simulink model "RobustLateralLPV"  (R2020b)
settings: Solver=VariableStepAuto  StartTime=0.0  StopTime=64  RelTol=1e-3
values from neighbouring files (symbols this model uses):
  A11 = [-(Cf + Cr)/(m*vxmax)        -vxmin + (Cr*Lr - Cf*Lf)/(m*vxmax) ... (first row only)    [Lab_Lateral.m]
  A12 = [-(Cf + Cr)/(m*vxmin)        -vxmin + (Cr*Lr - Cf*Lf)/(m*vxmin) ... (first row only)    [Lab_Lateral.m]
  A21 = [-(Cf + Cr)/(m*vxmax)        -vxmax + (Cr*Lr - Cf*Lf)/(m*vxmax) ... (first row only)    [Lab_Lateral.m]
  A22 = [-(Cf + Cr)/(m*vxmin)        -vxmax + (Cr*Lr - Cf*Lf)/(m*vxmin) ... (first row only)    [Lab_Lateral.m]
  B = [Cf/m; Lf*Cf/Iz]    [Lab_Lateral.m]
  C = [0 1]    [Lab_Lateral.m]
  D = [0]    [Lab_Lateral.m]
  listG = {G1, G2, G3, G4}    [H_inf_control_designLPV.m]
  listK = {K1, K2, K3, K4}    [H_inf_control_designLPV.m]
  m = 1621    [Lab_Lateral.m]
  rho1Max = vxmax    (= 15)    [Lab_Lateral.m]
  rho1Min = vxmin    (= 5)    [Lab_Lateral.m]
  rho2Max = 1/vxmin    (= 0.2)    [Lab_Lateral.m]
  rho2Min = 1/vxmax    (= 0.0666666666667)    [Lab_Lateral.m]
libraries: simulink x4, cstblocks x1
settings Model: Creator=DELL  LastModifiedBy=DELL

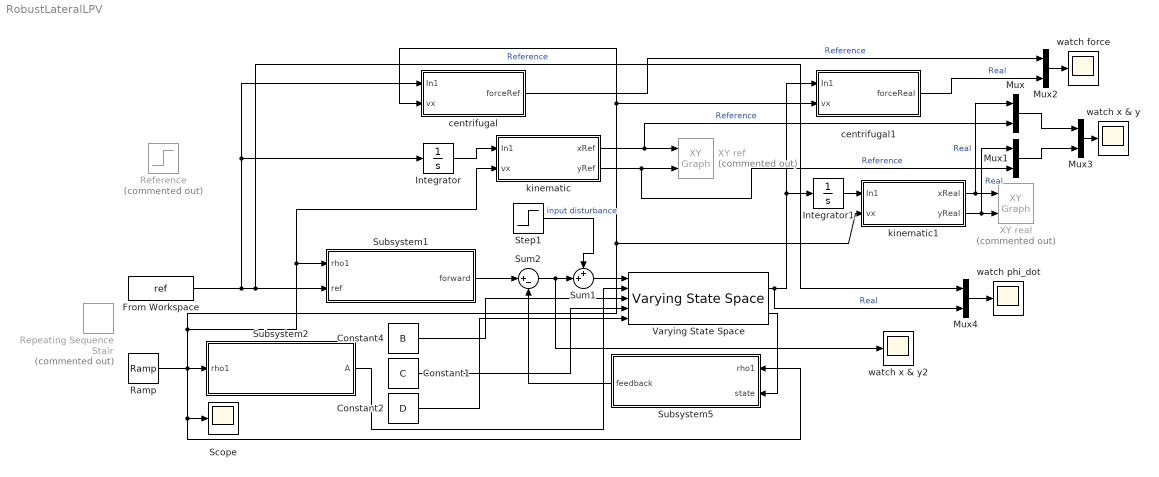
== system RobustLateralLPV ==
  Constant1 : Constant  Value=C  VectorParams1D=off
  Constant2 : Constant  Value=D
  Constant4 : Constant  Value=B
  From Workspace : FromWorkspace  VariableName=ref
  Integrator : Integrator
  Integrator1 : Integrator
  Mux{,1..4} (5 alike) : Mux  Inputs=2
  Ramp : simulink/Sources/Ramp  slope=0.2  start=20  InitialOutput=5
  Reference : Step  Commented=on  SampleTime=0
  Repeating Sequence Stair : simulink/Sources/Repeating Sequence Stair  Commented=on  OutValues=[5 11 15 9 7 5].'  tsamp=10  OutMin=[]  OutMax=[]  OutDataTypeStr=double  OutputDataTypeScalingMode=double  OutDataType=fixdt(0,8)  ConRadixGroup=Best Precision: Vector-wise  OutScaling=2^-12
  Scope : Scope
  Step1 : Step  Time=2  After=0.02*0  SampleTime=0
  Subsystem1 : Subsystem
  Subsystem2 : Subsystem
  Subsystem5 : Subsystem
  Sum1 : Sum  Inputs=++|
  Sum2 : Sum  Inputs=|+-
  Varying State Space : cstblocks/Linear Parameter Varying/Varying State Space  x0=0  xNames=''  OutputX=on  OutputDX=off
  XY real : simulink/Sinks/XY Graph  Commented=on  xmin=0  xmax=400  ymin=0  ymax=350  st=ts
  XY ref : simulink/Sinks/XY Graph  Commented=on  xmin=0  xmax=400  ymin=0  ymax=350  st=ts
  centrifugal : Subsystem
  centrifugal1 : Subsystem
  kinematic : Subsystem
  kinematic1 : Subsystem
  watch force : Scope
  watch phi_dot : Scope
  watch x & y : Scope
  watch x & y2 : Scope
  wires:
  Sum1/1 -> Varying State Space/1
  Mux/1 -> Mux3/1
  kinematic/1(xRef) -> Mux/2, XY ref/1  "Reference"
  Integrator/1 -> kinematic/1(In1)
  Integrator1/1 -> kinematic1/1(In1)
  Varying State Space/1 -> Mux4/2, centrifugal1/1(In1), Integrator1/1  "Real"
  centrifugal1/1(forceReal) -> Mux2/2  "Real"
  Sum2/1 -> watch x & y2/1, Sum1/2
  kinematic/2(yRef) -> Mux1/2, XY ref/2  "Reference"
  Step1/1 -> Sum1/1  "input disturbance"
  kinematic1/2(yReal) -> Mux1/1, XY real/2  "Real"
  centrifugal/1(forceRef) -> Mux2/1  "Reference"
  kinematic1/1(xReal) -> Mux/1, XY real/1  "Real"
  Subsystem1/1(forward) -> Sum2/1
  Subsystem5/1(feedback) -> Sum2/2
  Mux1/1 -> Mux3/2
  From Workspace/1 -> centrifugal/1(In1), Integrator/1, Mux4/1, Subsystem1/2(ref)  "Reference"
  Varying State Space/2 -> Subsystem5/2(state)
  Constant4/1 -> Varying State Space/3
  Constant1/1 -> Varying State Space/4
  Constant2/1 -> Varying State Space/5
  Ramp/1 -> Subsystem2/1(rho1), kinematic/2(vx), Subsystem1/1(rho1), centrifugal/2(vx), centrifugal1/2(vx), kinematic1/2(vx), Subsystem5/1(rho1), Scope/1
  Subsystem2/1(A) -> Varying State Space/2
  Mux4/1 -> watch phi_dot/1
  Mux3/1 -> watch x & y/1
  Mux2/1 -> watch force/1

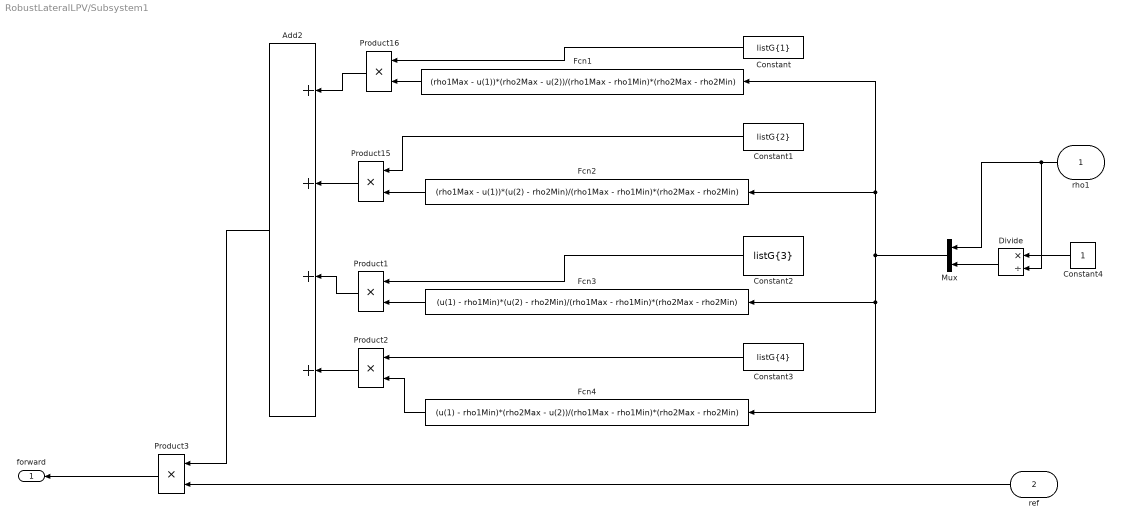
== system RobustLateralLPV/Subsystem1 ==
  rho1 : Inport
  ref : Inport  Port=2
  Add2 : Sum  Inputs=++++
  Constant : Constant  Value=listG{1}
  Constant1 : Constant  Value=listG{2}
  Constant2 : Constant  Value=listG{3}
  Constant3 : Constant  Value=listG{4}
  Constant4 : Constant
  Divide : Product  Inputs=*/
  Fcn1 : Fcn  Expr=(rho1Max - u(1))*(rho2Max - u(2))/(rho1Max - rho1Min)*(rho2Max - rho2Min)
  Fcn2 : Fcn  Expr=(rho1Max - u(1))*(u(2) - rho2Min)/(rho1Max - rho1Min)*(rho2Max - rho2Min)
  Fcn3 : Fcn  Expr=(u(1) - rho1Min)*(u(2) - rho2Min)/(rho1Max - rho1Min)*(rho2Max - rho2Min)
  Fcn4 : Fcn  Expr=(u(1) - rho1Min)*(rho2Max - u(2))/(rho1Max - rho1Min)*(rho2Max - rho2Min)
  Mux : Mux  Inputs=2
  Product{1..3,15..16} (5 alike) : Product  RndMeth=Zero
  forward : Outport  VectorParamsAs1DForOutWhenUnconnected=off
  wires:
  Fcn1/1 -> Product16/2
  Fcn2/1 -> Product15/2
  Product16/1 -> Add2/1
  Product15/1 -> Add2/2
  Constant1/1 -> Product15/1
  Constant/1 -> Product16/1
  rho1/1 -> Divide/2, Mux/1
  Mux/1 -> Fcn4/1, Fcn3/1, Fcn1/1, Fcn2/1
  Fcn3/1 -> Product1/2
  Constant2/1 -> Product1/1
  Product1/1 -> Add2/3
  Product2/1 -> Add2/4
  Fcn4/1 -> Product2/2
  Constant3/1 -> Product2/1
  Product3/1 -> forward/1
  Add2/1 -> Product3/1
  ref/1 -> Product3/2
  Divide/1 -> Mux/2
  Constant4/1 -> Divide/1

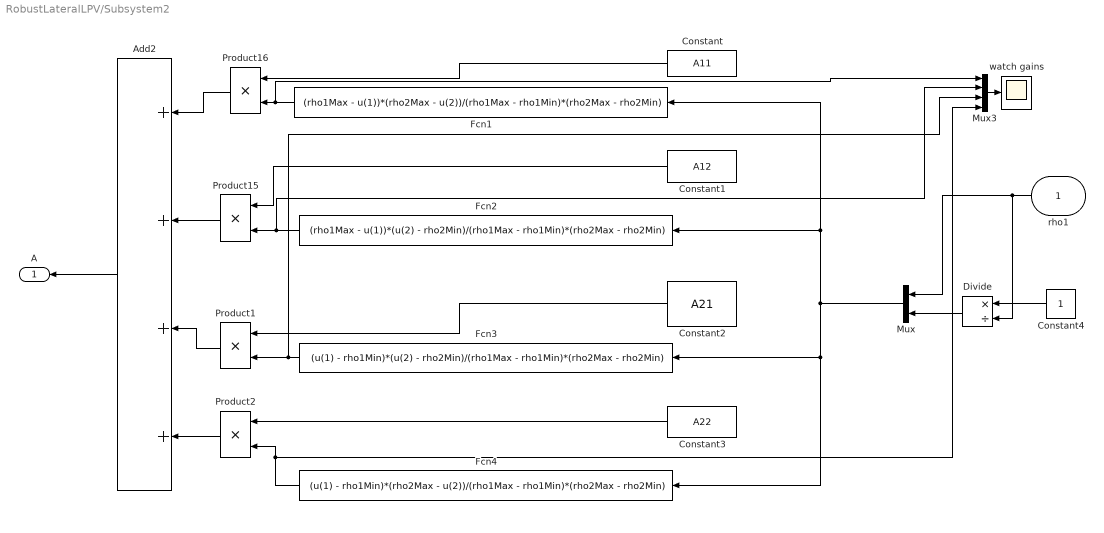
== system RobustLateralLPV/Subsystem2 ==
  rho1 : Inport
  Add2 : Sum  Inputs=++++
  Constant : Constant  Value=A11
  Constant1 : Constant  Value=A12
  Constant2 : Constant  Value=A21
  Constant3 : Constant  Value=A22
  Constant4 : Constant
  Divide : Product  Inputs=*/
  Fcn1 : Fcn  Expr=(rho1Max - u(1))*(rho2Max - u(2))/(rho1Max - rho1Min)*(rho2Max - rho2Min)
  Fcn2 : Fcn  Expr=(rho1Max - u(1))*(u(2) - rho2Min)/(rho1Max - rho1Min)*(rho2Max - rho2Min)
  Fcn3 : Fcn  Expr=(u(1) - rho1Min)*(u(2) - rho2Min)/(rho1Max - rho1Min)*(rho2Max - rho2Min)
  Fcn4 : Fcn  Expr=(u(1) - rho1Min)*(rho2Max - u(2))/(rho1Max - rho1Min)*(rho2Max - rho2Min)
  Mux : Mux  Inputs=2
  Mux3 : Mux
  Product{1..2,15..16} (4 alike) : Product  RndMeth=Zero
  watch gains : Scope
  A : Outport  VectorParamsAs1DForOutWhenUnconnected=off
  wires:
  Fcn1/1 -> Mux3/1, Product16/2
  Fcn2/1 -> Mux3/2, Product15/2
  Product15/1 -> Add2/2
  Constant1/1 -> Product15/1
  Constant/1 -> Product16/1
  rho1/1 -> Divide/2, Mux/1
  Mux/1 -> Fcn4/1, Fcn3/1, Fcn1/1, Fcn2/1
  Constant2/1 -> Product1/1
  Product1/1 -> Add2/3
  Product2/1 -> Add2/4
  Fcn4/1 -> Mux3/4, Product2/2
  Constant3/1 -> Product2/1
  Divide/1 -> Mux/2
  Constant4/1 -> Divide/1
  Add2/1 -> A/1
  Mux3/1 -> watch gains/1
  Fcn3/1 -> Product1/2, Mux3/3
  Product16/1 -> Add2/1

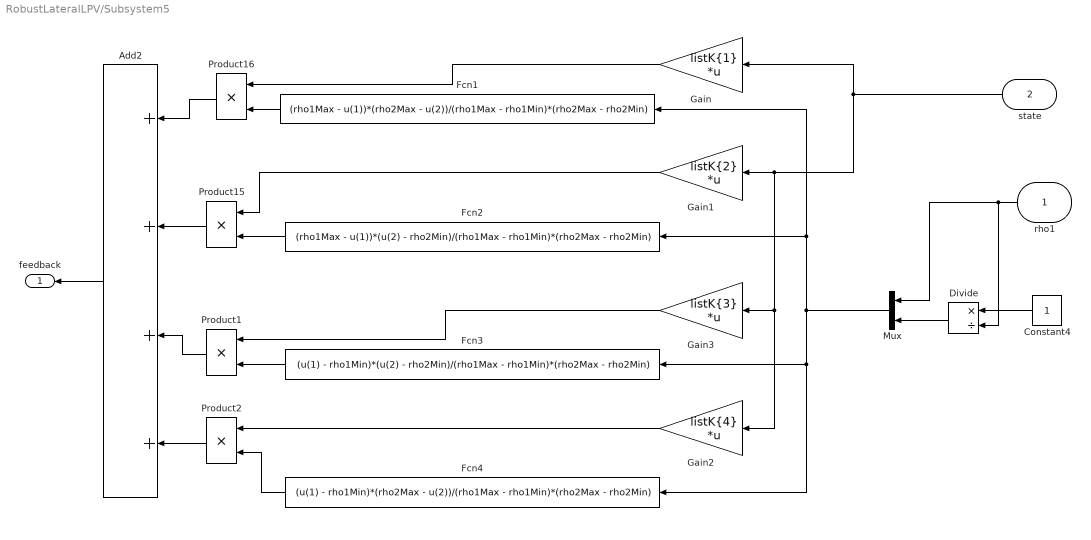
== system RobustLateralLPV/Subsystem5 ==
  rho1 : Inport
  state : Inport  Port=2
  Add2 : Sum  Inputs=++++
  Constant4 : Constant
  Divide : Product  Inputs=*/
  Fcn1 : Fcn  Expr=(rho1Max - u(1))*(rho2Max - u(2))/(rho1Max - rho1Min)*(rho2Max - rho2Min)
  Fcn2 : Fcn  Expr=(rho1Max - u(1))*(u(2) - rho2Min)/(rho1Max - rho1Min)*(rho2Max - rho2Min)
  Fcn3 : Fcn  Expr=(u(1) - rho1Min)*(u(2) - rho2Min)/(rho1Max - rho1Min)*(rho2Max - rho2Min)
  Fcn4 : Fcn  Expr=(u(1) - rho1Min)*(rho2Max - u(2))/(rho1Max - rho1Min)*(rho2Max - rho2Min)
  Gain : Gain  Gain=listK{1}  Multiplication=Matrix(K*u) (u vector)
  Gain1 : Gain  Gain=listK{2}  Multiplication=Matrix(K*u) (u vector)
  Gain2 : Gain  Gain=listK{4}  Multiplication=Matrix(K*u) (u vector)
  Gain3 : Gain  Gain=listK{3}  Multiplication=Matrix(K*u) (u vector)
  Mux : Mux  Inputs=2
  Product{1..2,15..16} (4 alike) : Product  RndMeth=Zero
  feedback : Outport  VectorParamsAs1DForOutWhenUnconnected=off
  wires:
  Fcn1/1 -> Product16/2
  Fcn2/1 -> Product15/2
  Product16/1 -> Add2/1
  Product15/1 -> Add2/2
  Gain1/1 -> Product15/1
  Gain/1 -> Product16/1
  rho1/1 -> Divide/2, Mux/1
  Mux/1 -> Fcn4/1, Fcn3/1, Fcn1/1, Fcn2/1
  Fcn3/1 -> Product1/2
  Gain3/1 -> Product1/1
  Product1/1 -> Add2/3
  Product2/1 -> Add2/4
  Fcn4/1 -> Product2/2
  Gain2/1 -> Product2/1
  Add2/1 -> feedback/1
  Divide/1 -> Mux/2
  Constant4/1 -> Divide/1
  state/1 -> Gain2/1, Gain3/1, Gain1/1, Gain/1

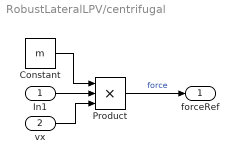
== system RobustLateralLPV/centrifugal ==
  In1 : Inport
  vx : Inport  Port=2
  Constant : Constant  Value=m
  Product : Product  Inputs=3
  forceRef : Outport
  wires:
  In1/1 -> Product/2
  Constant/1 -> Product/1
  Product/1 -> forceRef/1  "force"
  vx/1 -> Product/3

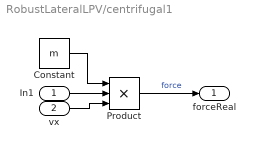
== system RobustLateralLPV/centrifugal1 ==
  In1 : Inport
  vx : Inport  Port=2
  Constant : Constant  Value=m
  Product : Product  Inputs=3
  forceReal : Outport
  wires:
  In1/1 -> Product/2
  Constant/1 -> Product/1
  Product/1 -> forceReal/1  "force"
  vx/1 -> Product/3

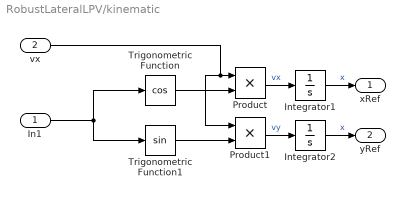
== system RobustLateralLPV/kinematic ==
  In1 : Inport
  vx : Inport  Port=2
  Integrator1 : Integrator
  Integrator2 : Integrator
  Product : Product
  Product1 : Product
  Trigonometric Function : Trigonometry  Operator=cos
  Trigonometric Function1 : Trigonometry
  xRef : Outport
  yRef : Outport  Port=2
  wires:
  In1/1 -> Trigonometric Function1/1, Trigonometric Function/1
  Trigonometric Function1/1 -> Product1/2
  Trigonometric Function/1 -> Product/2
  vx/1 -> Product1/1, Product/1
  Product/1 -> Integrator1/1  "vx"
  Integrator1/1 -> xRef/1  "x"
  Product1/1 -> Integrator2/1  "vy"
  Integrator2/1 -> yRef/1  "x"

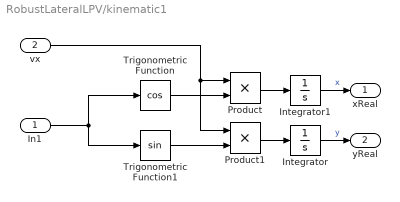
== system RobustLateralLPV/kinematic1 ==
  In1 : Inport
  vx : Inport  Port=2
  Integrator : Integrator
  Integrator1 : Integrator
  Product : Product
  Product1 : Product
  Trigonometric Function : Trigonometry  Operator=cos
  Trigonometric Function1 : Trigonometry
  xReal : Outport
  yReal : Outport  Port=2
  wires:
  In1/1 -> Trigonometric Function1/1, Trigonometric Function/1
  Trigonometric Function1/1 -> Product1/2
  Trigonometric Function/1 -> Product/2
  vx/1 -> Product1/1, Product/1
  Product/1 -> Integrator1/1
  Integrator1/1 -> xReal/1  "x"
  Product1/1 -> Integrator/1
  Integrator/1 -> yReal/1  "y"
